simulink model "ODE_Hand_Model_v02"  (Simulink 7.5)
settings: Solver=ode1  StartTime=0.0  StopTime=inf  FixedStep=0.0315/3  RelTol=1e-3
settings Model: Creator=nihil  LastModifiedBy=konstantinos

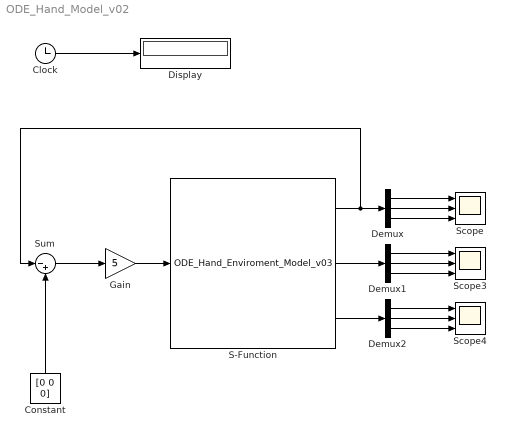
== system ODE_Hand_Model_v02 ==
  Clock : Clock
      settings: Decimation=10
  Constant : Constant  Value=[0 0 0]  OutDataType=fixdt(1, 16)  OutScaling=2^0
  Demux : Demux  Outputs=3
  Demux1 : Demux  Outputs=3
  Demux2 : Demux  Outputs=3
  Display : Display
  Gain : Gain  Gain=5  ParameterDataType=fixdt(1, 16)  ParameterScaling=2^0  OutDataType=fixdt(1, 16)  OutScaling=2^0
  S-Function : S-Function  FunctionName=ODE_Hand_Enviroment_Model_v03  EnableBusSupport=off
  Scope : Scope  NumInputPorts=3
      settings: TimeRange=0.5  YMin=-0.005~-5~-5  YMax=0.105~5~5
  Scope3 : Scope  NumInputPorts=3
      settings: YMin=-0.005~-5~-5  YMax=0.105~5~5  SaveName=ScopeData3
  Scope4 : Scope  NumInputPorts=3
      settings: YMin=-0.005~-5~-5  YMax=0.105~5~5  SaveName=ScopeData4
  Sum : Sum  Inputs=|-+  OutDataType=fixdt(1, 16)  OutScaling=2^0
  wires:
  Clock/1 -> Display/1
  Constant/1 -> Sum/2
  S-Function/1 -> Demux/1, Sum/1
  S-Function/2 -> Demux1/1
  S-Function/3 -> Demux2/1
  Demux/1 -> Scope/1
  Demux/2 -> Scope/2
  Demux/3 -> Scope/3
  Demux1/1 -> Scope3/1
  Demux1/2 -> Scope3/2
  Demux1/3 -> Scope3/3
  Demux2/1 -> Scope4/1
  Demux2/2 -> Scope4/2
  Demux2/3 -> Scope4/3
  Sum/1 -> Gain/1
  Gain/1 -> S-Function/1
